simulink model "es5_sim"  (Simulink 7.9)
settings: Solver=ode45  StartTime=0.0  StopTime=10  RelTol=1e-3
values from neighbouring files (symbols this model uses):
  A = [-1 -5;7 -2]    [es5.m]
  B = [1 0]'    [es5.m]
  C = [1 1]    [es5.m]
  L = place(A',C',aval_oss)'    [es5.m]
  X0 = [5 5]    [es5.m]
undefined symbols (not defined in the file or in its folder): K
settings Model: Creator=claudio  LastModifiedBy=patrizio
settings OptimizationCC: InlineInvariantSignals=on  InitFltsAndDblsToZero=on
settings DebuggingCC: SaveWithParameterizedLinksMsg=none  SignalResolutionControl=TryResolveAllWithWarning  MultiTaskDSMMsg=warning  MultiTaskCondExecSysMsg=none  FcnCallInpInsideContextMsg=Use local settings  StrictBusMsg=None
settings RTWCC: IncludeERTFirstTime=on
settings GRTTargetCC: TargetFcnLib=ansi_tfl_tmw.mat  CombineOutputUpdateFcns=off  GRTInterface=on

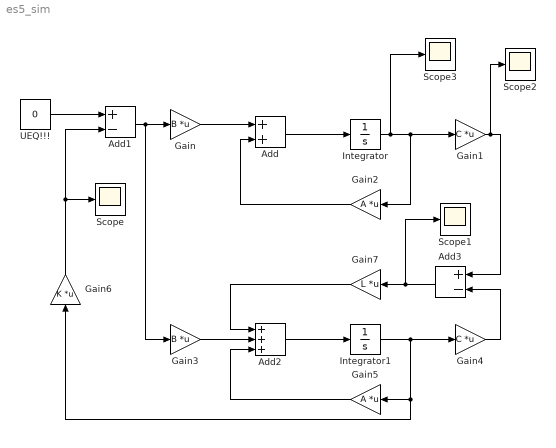
== system es5_sim ==
  Add : Sum
  Add1 : Sum  Inputs=+-
  Add2 : Sum  Inputs=+++
  Add3 : Sum  Inputs=+-
  Gain : Gain  Gain=B  Multiplication=Matrix(K*u)
  Gain1 : Gain  Gain=C  Multiplication=Matrix(K*u)
  Gain2 : Gain  Gain=A  Multiplication=Matrix(K*u)
  Gain3 : Gain  Gain=B  Multiplication=Matrix(K*u)
  Gain4 : Gain  Gain=C  Multiplication=Matrix(K*u)
  Gain5 : Gain  Gain=A  Multiplication=Matrix(K*u)
  Gain6 : Gain  Gain=K  Multiplication=Matrix(K*u)
  Gain7 : Gain  Gain=L  Multiplication=Matrix(K*u)
  Integrator : Integrator  InitialCondition=X0
  Integrator1 : Integrator
  Scope{,1..3} (4 alike) : Scope
      Scope2 settings: SaveName=ScopeData2
      Scope3 settings: SaveName=ScopeData3
  UEQ!!! : Constant  Value=0
  wires:
  Integrator/1 -> Gain1/1, Gain2/1, Scope3/1
  Add/1 -> Integrator/1
  Gain2/1 -> Add/2
  Gain/1 -> Add/1
  Add1/1 -> Gain/1, Gain3/1
  Integrator1/1 -> Gain4/1, Gain5/1, Gain6/1
  Add2/1 -> Integrator1/1
  Gain6/1 -> Add1/2, Scope/1
  Gain4/1 -> Add3/2
  Gain1/1 -> Add3/1, Scope2/1
  Add3/1 -> Gain7/1, Scope1/1
  Gain7/1 -> Add2/1
  Gain3/1 -> Add2/2
  Gain5/1 -> Add2/3
  UEQ!!!/1 -> Add1/1
